simulink library "ForcesExterieures"  (R2018a)
settings: Solver=VariableStepAuto  StartTime=0.0  StopTime=10.0  RelTol=1e-3
values from neighbouring files (symbols this model uses):
  c_dist_int = (0:1:1999)    [UntitFSDAFled.m]
undefined symbols (not defined in the file or in its folder): alphaCorr_int
settings Model: Creator=thomas.moser  LastModifiedBy=thomas.moser

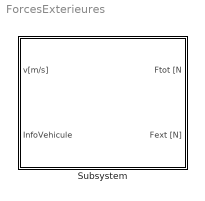
== system ForcesExterieures ==
  Subsystem : Subsystem  mask{rho=1.225, g=9.81}
      mask prompts: rho "Densité de l'air [kg/m^3] :"; g "Accélération gravitationelle [m/s^2] :"

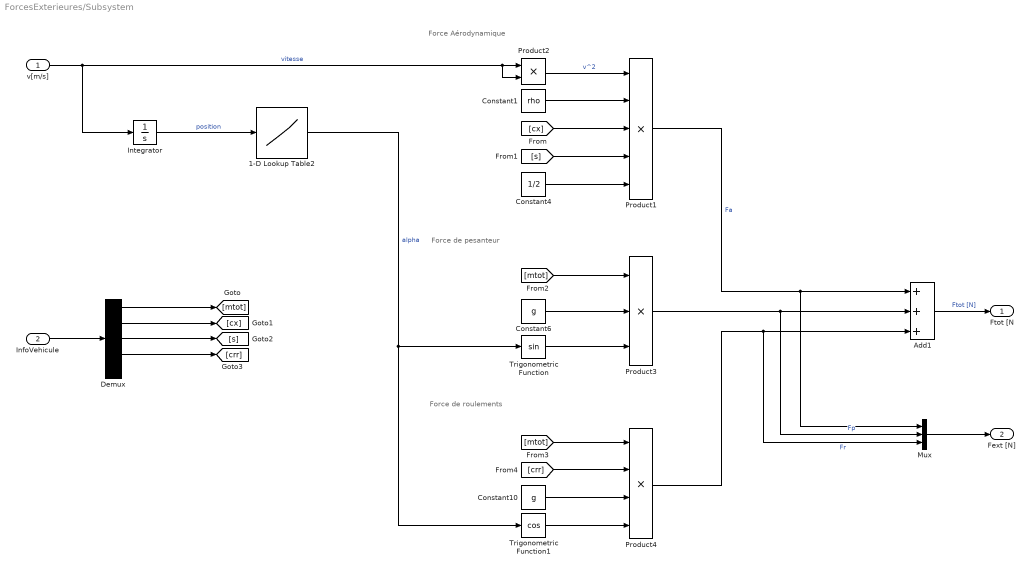
== system ForcesExterieures/Subsystem ==
  note: Force de pesanteur
  note: Force de roulements
  note: Force Aérodynamique
  v[m/s] : Inport
  InfoVehicule : Inport  Port=2
  1-D Lookup Table2 : Lookup_n-D  NumberOfTableDimensions=1  BreakpointsForDimension1=c_dist_int(1:1:length(c_dist_int)-1)  Table=alphaCorr_int  InternalRulePriority=Speed  RndMeth=Simplest  InputSameDT=on
  Add1 : Sum  Inputs=+++
  Constant1 : Constant  Value=rho
  Constant10 : Constant  Value=g
  Constant4 : Constant  Value=1/2
  Constant6 : Constant  Value=g
  Demux : Demux  Outputs=5
  Integrator : Integrator
  Mux : Mux  Inputs=3
  Product1 : Product  Inputs=5
  Product2 : Product
  Product3 : Product  Inputs=3
  Product4 : Product  Inputs=4
  Trigonometric Function : Trigonometry
  Trigonometric Function1 : Trigonometry  Operator=cos
  Ftot [N : Outport
  Fext [N] : Outport  Port=2
  wires:
  Constant1/1 -> Product1/2
  1-D Lookup Table2/1 -> Trigonometric Function/1, Trigonometric Function1/1  "alpha"
  v[m/s]/1 -> Integrator/1, Product2/2, Product2/1  "vitesse"
  Add1/1 -> Ftot [N/1  "Ftot [N]"
  Product4/1 -> Mux/3, Add1/3  "Fr"
  Constant4/1 -> Product1/5
  Constant6/1 -> Product3/2
  Constant10/1 -> Product4/3
  Product3/1 -> Mux/2, Add1/2  "Fp"
  Product2/1 -> Product1/1  "v^2"
  Product1/1 -> Mux/1, Add1/1  "Fa"
  Trigonometric Function1/1 -> Product4/4
  Trigonometric Function/1 -> Product3/3
  InfoVehicule/1 -> Demux/1
  Mux/1 -> Fext [N]/1
  Integrator/1 -> 1-D Lookup Table2/1  "position"
  Demux/1 -> [mtot]
  Demux/2 -> [cx]
  Demux/4 -> [crr]
  Demux/3 -> [s]
  [cx] -> Product1/3
  [s] -> Product1/4
  [mtot] -> Product3/1
  [mtot] -> Product4/1
  [crr] -> Product4/2
